simulink model "Open_loop_rotor_flux_observer"  (R2021a)
settings: Solver=VariableStepAuto  StartTime=0.0  StopTime=10.0  RelTol=1e-3
settings Model: Creator=Mehra  LastModifiedBy=Mehra

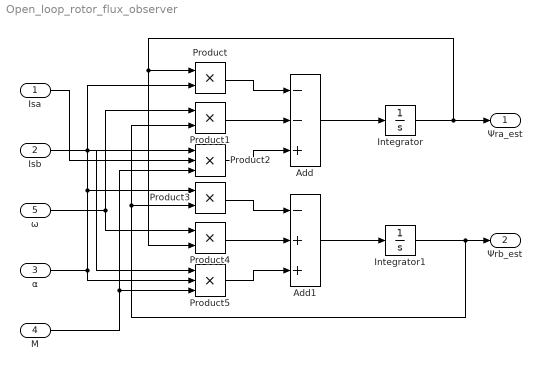
== system Open_loop_rotor_flux_observer ==
  Isa : Inport
  Isb : Inport  Port=2
  α : Inport  Port=3
  M : Inport  Port=4
  ω : Inport  Port=5
  Add : Sum  Inputs=--+
  Add1 : Sum  Inputs=-++
  Integrator : Integrator
  Integrator1 : Integrator
  Product{,1,3..4} (4 alike) : Product
  Product2 : Product  Inputs=3
  Product5 : Product  Inputs=3
  Ψra_est : Outport
  Ψrb_est : Outport  Port=2
  wires:
  Product/1 -> Add/1
  Product1/1 -> Add/2
  Product2/1 -> Add/3
  Product3/1 -> Add1/1
  Product4/1 -> Add1/2
  Product5/1 -> Add1/3
  Add/1 -> Integrator/1
  Integrator/1 -> Product/1, Product4/2, Ψra_est/1
  α/1 -> Product5/2, Product2/1, Product/2, Product3/1
  ω/1 -> Product4/1, Product1/1
  Add1/1 -> Integrator1/1
  Integrator1/1 -> Product1/2, Product3/2, Ψrb_est/1
  Isa/1 -> Product2/2
  M/1 -> Product5/3, Product2/3
  Isb/1 -> Product5/1
